simulink model "ModelAided_PAHRS"  (R2025b)
settings: Solver=ode4  StartTime=0.0  StopTime=300  RelTol=1e-3
values from neighbouring files (symbols this model uses):
  b_a = [0.090; -0.120; 0.075]    [Initilization.m]
  b_w = [-0.0009; 0.0010; -0.0015]    [Initilization.m]
  M_a = [50000, -15000, 10000;                   -7500, -60000, 12500;                  -12500,   5000, 20000] * 1E-6    [Initilization.m]
  M_w = [40000, -14000,  12500;                       0, -30000,  -7500;                       0,      0, -17500] * 1E-6    [Initilization.m]
libraries: slpidlib x16, simulink_extras x13, simulink x8, aerolibobsolete x4
(part 1 of 3)
settings Model: Creator=Arsinsoft  LastModifiedBy=Arsinsoft
settings OptimizationCC: ReuseModelBlockBuffer=off
settings RTWCC: GPUComputeCapability=3.5

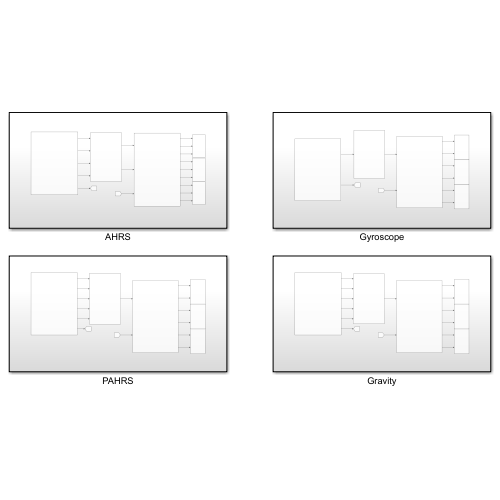
[thumbnail: Simulink's stored preview of the top-level diagram]
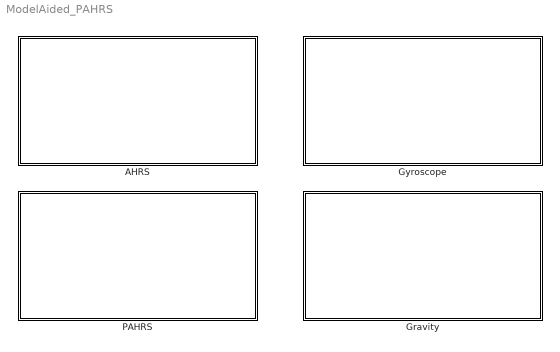
== system ModelAided_PAHRS ==
  AHRS : Subsystem
  Gravity : Subsystem
  Gyroscope : Subsystem
  PAHRS : Subsystem

== system ModelAided_PAHRS/AHRS ==
  AHRS (Euler - KF - Closed Loop) : Subsystem
  Dynamic Model : Subsystem
  Scope : Subsystem
  Scope1 : Scope  NumInputPorts=3
      settings: ActiveDisplayYMinimum=-4.56009  ActiveDisplayYMaximum=22.67075
  Scope2 : Scope  NumInputPorts=3
      settings: ActiveDisplayYMinimum=-2.66951  ActiveDisplayYMaximum=2.86704
  Scope3 : Scope  NumInputPorts=3
      settings: ActiveDisplayYMinimum=-8.24822  ActiveDisplayYMaximum=24.22827  DataLoggingVariableName=ScopeData2
  wires:
  Dynamic Model/4(psi_mes) -> AHRS (Euler - KF - Closed Loop)/4(psi_mes)
  Dynamic Model/3(a_B) -> AHRS (Euler - KF - Closed Loop)/3(a_B)
  Dynamic Model/2(f_B) -> AHRS (Euler - KF - Closed Loop)/2(f_B)
  Dynamic Model/1(omega_B) -> AHRS (Euler - KF - Closed Loop)/1(omega_B)
  AHRS (Euler - KF - Closed Loop)/1(xhat) -> Scope/1(xhat)
  AHRS (Euler - KF - Closed Loop)/2(y_mes) -> Scope/2(y_mes)
  Scope/1(phi_true) -> Scope1/1  "phi_true"
  Scope/2(phi_mes) -> Scope1/2  "phi_mes"
  Scope/3(phi_hat) -> Scope1/3  "phi_hat"
  Scope/5(theta_mes) -> Scope2/2  "theta_mes"
  Scope/4(theta_true) -> Scope2/1  "theta_true"
  Scope/6(theta_hat) -> Scope2/3  "theta_hat"
  Scope/7(psi_true) -> Scope3/1  "psi_true"
  Scope/8(psi_mes) -> Scope3/2  "psi_mes"
  Scope/9(psi_hat) -> Scope3/3  "psi_hat"
  Dynamic Model/5(A_true) -> [A_true]
  [A_true] -> Scope/3(A_true)

== system ModelAided_PAHRS/Gravity ==
  Dynamic Model : Subsystem
  PAHRS (Euler - KF - Closed Loop) : Subsystem
  Scope : Subsystem
  Scope1 : Scope  NumInputPorts=2
      settings: ActiveDisplayYMinimum=-22.604189397145177  ActiveDisplayYMaximum=33.93959392130872
  Scope2 : Scope  NumInputPorts=2
      settings: ActiveDisplayYMinimum=-1.1950277273773284  ActiveDisplayYMaximum=1.0982346892038803  DataLoggingVariableName=ScopeData4
  Scope3 : Scope  NumInputPorts=2
      settings: ActiveDisplayYMinimum=-16.246693349234917  ActiveDisplayYMaximum=108.31140694961906  DataLoggingVariableName=ScopeData3
  wires:
  Scope/6(psi_gravity) -> Scope3/2  "psi_gravity"
  PAHRS (Euler - KF - Closed Loop)/1(xhat) -> Scope/1(xhat)
  Scope/1(phi_true) -> Scope1/1  "phi_true"
  Scope/2(phi_gravity) -> Scope1/2  "phi_gravity"
  Scope/3(theta_true) -> Scope2/1  "theta_true"
  Scope/4(theta_gravity) -> Scope2/2  "theta_gravity"
  Scope/5(psi_true) -> Scope3/1  "psi_true"
  [A_true] -> Scope/2(A_true)
  Dynamic Model/6(A_true) -> [A_true]
  Dynamic Model/5(psi_mes2) -> PAHRS (Euler - KF - Closed Loop)/5(psi_mes2)
  Dynamic Model/4(psi_mes1) -> PAHRS (Euler - KF - Closed Loop)/4(psi_mes1)
  Dynamic Model/3(a_B) -> PAHRS (Euler - KF - Closed Loop)/3(a_B)
  Dynamic Model/1(omega_B) -> PAHRS (Euler - KF - Closed Loop)/1(omega_B)
  Dynamic Model/2(f_B) -> PAHRS (Euler - KF - Closed Loop)/2(f_B)

== system ModelAided_PAHRS/Gyroscope ==
  Dynamic Model : Subsystem
  Propagation : Subsystem
  Scope : Subsystem
  Scope1 : Scope  NumInputPorts=2
      settings: ActiveDisplayYMinimum=-37.126063824866776  ActiveDisplayYMaximum=33.465463609284008
  Scope2 : Scope  NumInputPorts=2
      settings: ActiveDisplayYMinimum=-7.2234114605205  ActiveDisplayYMaximum=39.031362224782178  DataLoggingVariableName=ScopeData4
  Scope3 : Scope  NumInputPorts=2
      settings: ActiveDisplayYMinimum=-34.052279453447049  ActiveDisplayYMaximum=109.90874054758552  DataLoggingVariableName=ScopeData3
  wires:
  [A_true] -> Scope/2(A_true)
  Scope/5(psi_true) -> Scope3/1  "psi_true"
  Scope/4(theta_gyro) -> Scope2/2  "theta_gyro"
  Scope/3(theta_true) -> Scope2/1  "theta_true"
  Scope/2(phi_gyro) -> Scope1/2  "phi_gyro"
  Scope/1(phi_true) -> Scope1/1  "phi_true"
  Propagation/1(x_gyro) -> Scope/1(x_gyro)
  Scope/6(psi_gyro) -> Scope3/2  "psi_gyro"
  Dynamic Model/1(omega_B) -> Propagation/1(omega_B)
  Dynamic Model/2(A_true) -> [A_true]

== system ModelAided_PAHRS/PAHRS ==
  Dynamic Model : Subsystem
  PAHRS (Euler - KF - Closed Loop) : Subsystem
  Scope : Subsystem
  Scope1 : Scope  NumInputPorts=2
      settings: ActiveDisplayYMinimum=-6.9171932251670389  ActiveDisplayYMaximum=31.887881688968882
  Scope2 : Scope  NumInputPorts=2
      settings: ActiveDisplayYMinimum=-1.1472184157024201  ActiveDisplayYMaximum=1.0928796557242522  DataLoggingVariableName=ScopeData4
  Scope3 : Scope  NumInputPorts=2
      settings: ActiveDisplayYMinimum=-16.332769192632206  ActiveDisplayYMaximum=108.42060570484539  DataLoggingVariableName=ScopeData3
  wires:
  [A_true] -> Scope/2(A_true)
  Scope/5(psi_true) -> Scope3/1  "psi_true"
  Scope/4(theta_hat) -> Scope2/2  "theta_hat"
  Scope/3(theta_true) -> Scope2/1  "theta_true"
  Scope/2(phi_hat) -> Scope1/2  "phi_hat"
  Scope/1(phi_true) -> Scope1/1  "phi_true"
  PAHRS (Euler - KF - Closed Loop)/1(xhat) -> Scope/1(xhat)
  Scope/6(psi_hat) -> Scope3/2  "psi_hat"
  Dynamic Model/6(A_true) -> [A_true]
  Dynamic Model/5(psi_mes2) -> PAHRS (Euler - KF - Closed Loop)/5(psi_mes2)
  Dynamic Model/4(psi_mes1) -> PAHRS (Euler - KF - Closed Loop)/4(psi_mes1)
  Dynamic Model/3(a_B) -> PAHRS (Euler - KF - Closed Loop)/3(a_B)
  Dynamic Model/2(f_B) -> PAHRS (Euler - KF - Closed Loop)/2(f_B)
  Dynamic Model/1(omega_B) -> PAHRS (Euler - KF - Closed Loop)/1(omega_B)

== system ModelAided_PAHRS/AHRS/AHRS (Euler - KF - Closed Loop) ==
  omega_B : Inport
  f_B : Inport  Port=2
  a_B : Inport  Port=3
  psi_mes : Inport  Port=4
  Clock : Clock
  Enable : MATLAB Function  TreatAsAtomicUnit=on
  KF : Subsystem  TreatAsAtomicUnit=on
  Measurement : Subsystem
  Propagation : Subsystem
  Sum : Sum  Inputs=++|
  xhat : Outport
  y_mes : Outport  Port=2
  wires:
  Propagation/1(x_prop) -> KF/2(x_prop), Sum/1  "x_prop"
  Measurement/1(y_mes) -> y_mes/1, KF/3(y_mes)  "y_mes"
  KF/1(deltaxhat) -> Sum/2
  Enable/1(enable) -> KF/Enable
  Sum/1 -> Propagation/2(xhat), xhat/1
  Clock/1 -> Enable/1(t)
  omega_B/1 -> KF/1(omega_B), Propagation/1(omega_B)
  f_B/1 -> Measurement/2(f_B)
  a_B/1 -> Measurement/1(a_B)
  psi_mes/1 -> Measurement/3(psi_mes)

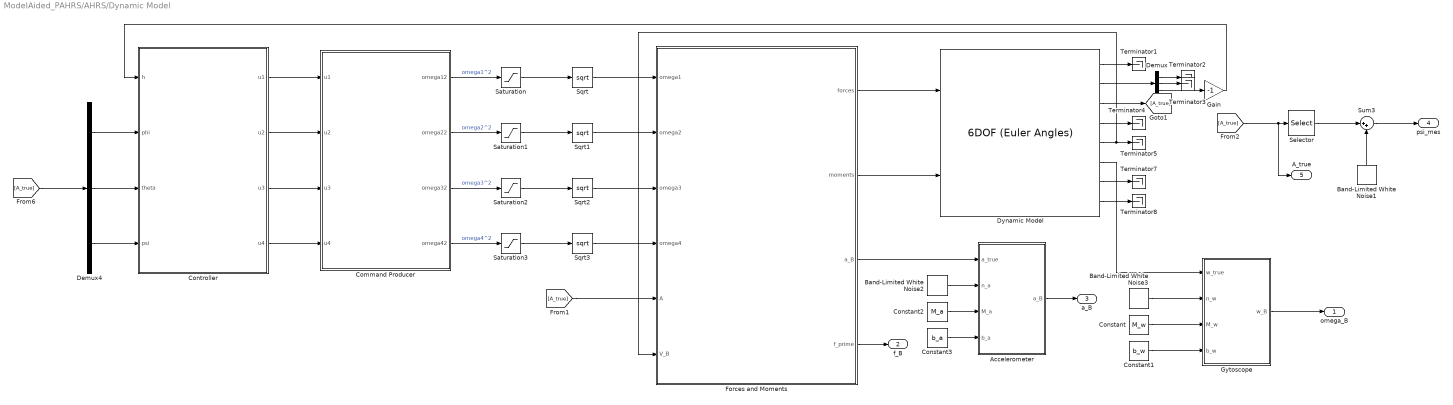
== system ModelAided_PAHRS/AHRS/Dynamic Model ==
  Accelerometer : MATLAB Function  TreatAsAtomicUnit=on
  Band-Limited White Noise1 : simulink/Sources/Band-Limited White Noise  Cov=1e-5  Ts=0.01  seed=[23341]
  Band-Limited White Noise2 : simulink/Sources/Band-Limited White Noise  Cov=1e-4  Ts=0.01  seed=[23341]
  Band-Limited White Noise3 : simulink/Sources/Band-Limited White Noise  Cov=1e-4  Ts=0.01  seed=[23341]
  Command Producer : MATLAB Function  TreatAsAtomicUnit=on
  Constant : Constant  Value=M_w
  Constant1 : Constant  Value=b_w
  Constant2 : Constant  Value=M_a
  Constant3 : Constant  Value=b_a
  Controller : Subsystem
  Demux : Demux  Outputs=3
  Demux4 : Demux  Outputs=3
  Dynamic Model : aerolibobsolete/6DOF (Euler Angles)  units=Metric (MKS)  mtype=Fixed  rep=Euler Angles  xme_0=[0 0 0]  Vm_0=[0 0 0]  eul_0=[0 0 0]  pm_0=[0 0 0]  mass_0=0.296  mass_e=0.5  mass_f=2.0  inertia=[0.0049, 0, 0; 0, 0.0049, 0; 0, 0, 0.0088]  inertia_e=eye(3)  inertia_f=2*eye(3)  k_quat=1.0  vre_flag=on  abi_flag=off  aMode=0  xme_statename=''  Vm_statename=''  eul_statename=''  quat_statename=''  pm_statename=''  mass_statename=''
  Forces and Moments : MATLAB Function  TreatAsAtomicUnit=on
  Gain : Gain  Gain=-1
  Gytoscope : MATLAB Function  TreatAsAtomicUnit=on
  Saturation{,1..3} (4 alike) : Saturate  UpperLimit=7e6  LowerLimit=138e3
  Selector : Selector  InputPortWidth=3  IndexOptions=Index vector (dialog)  Indices=[3]  OutputSizes=1
  Sqrt{,1..3} (4 alike) : Sqrt
  Sum3 : Sum  Inputs=|++
  Terminator{1..5,7..8} (7 alike) : Terminator
  omega_B : Outport
  f_B : Outport  Port=2
  a_B : Outport  Port=3
  psi_mes : Outport  Port=4
  A_true : Outport  Port=5
  wires:
  Forces and Moments/2(moments) -> Dynamic Model/2
  Forces and Moments/1(forces) -> Dynamic Model/1
  Sum3/1 -> psi_mes/1
  Dynamic Model/1 -> Terminator1/1
  Dynamic Model/3 -> [A_true]
  Dynamic Model/4 -> Terminator4/1
  Dynamic Model/7 -> Terminator7/1
  Dynamic Model/8 -> Terminator8/1
  Dynamic Model/5 -> Terminator5/1, Forces and Moments/6(V_B)
  Band-Limited White Noise1/1 -> Sum3/2
  Selector/1 -> Sum3/1
  [A_true] -> Forces and Moments/5(A)
  [A_true] -> A_true/1, Selector/1
  Dynamic Model/6 -> Gytoscope/1(w_true)
  [A_true] -> Demux4/1
  Demux4/3 -> Controller/4(psi)
  Demux4/2 -> Controller/3(theta)
  Demux4/1 -> Controller/2(phi)
  Command Producer/2(omega22) -> Saturation1/1  "omega2^2"
  Controller/1(u1) -> Command Producer/1(u1)
  Controller/3(u3) -> Command Producer/3(u3)
  Command Producer/4(omega42) -> Saturation3/1  "omega4^2"
  Saturation/1 -> Sqrt/1
  Controller/4(u4) -> Command Producer/4(u4)
  Saturation3/1 -> Sqrt3/1
  Command Producer/1(omega12) -> Saturation/1  "omega1^2"
  Command Producer/3(omega32) -> Saturation2/1  "omega3^2"
  Saturation2/1 -> Sqrt2/1
  Controller/2(u2) -> Command Producer/2(u2)
  Saturation1/1 -> Sqrt1/1
  Sqrt/1 -> Forces and Moments/1(omega1)
  Sqrt1/1 -> Forces and Moments/2(omega2)
  Sqrt2/1 -> Forces and Moments/3(omega3)
  Sqrt3/1 -> Forces and Moments/4(omega4)
  Dynamic Model/2 -> Demux/1
  Demux/1 -> Terminator2/1
  Demux/2 -> Terminator3/1
  Demux/3 -> Gain/1
  Gain/1 -> Controller/1(h)
  Forces and Moments/4(f_prime) -> f_B/1
  Accelerometer/1(a_B) -> a_B/1
  Forces and Moments/3(a_B) -> Accelerometer/1(a_true)
  Band-Limited White Noise2/1 -> Accelerometer/2(n_a)
  Band-Limited White Noise3/1 -> Gytoscope/2(n_w)
  Gytoscope/1(w_B) -> omega_B/1
  Constant/1 -> Gytoscope/3(M_w)
  Constant1/1 -> Gytoscope/4(b_w)
  Constant3/1 -> Accelerometer/4(b_a)
  Constant2/1 -> Accelerometer/3(M_a)

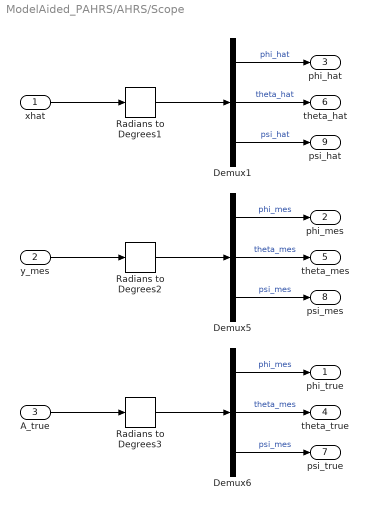
== system ModelAided_PAHRS/AHRS/Scope ==
  xhat : Inport
  y_mes : Inport  Port=2
  A_true : Inport  Port=3
  Demux1 : Demux  Outputs=3
  Demux5 : Demux  Outputs=3
  Demux6 : Demux  Outputs=3
  Radians to Degrees1 : simulink_extras/Transformations/Radians to Degrees
  Radians to Degrees2 : simulink_extras/Transformations/Radians to Degrees
  Radians to Degrees3 : simulink_extras/Transformations/Radians to Degrees
  phi_true : Outport
  phi_mes : Outport  Port=2
  phi_hat : Outport  Port=3
  theta_true : Outport  Port=4
  theta_mes : Outport  Port=5
  theta_hat : Outport  Port=6
  psi_true : Outport  Port=7
  psi_mes : Outport  Port=8
  psi_hat : Outport  Port=9
  wires:
  Demux1/2 -> theta_hat/1  "theta_hat"
  Demux1/3 -> psi_hat/1  "psi_hat"
  Demux1/1 -> phi_hat/1  "phi_hat"
  xhat/1 -> Radians to Degrees1/1
  Radians to Degrees1/1 -> Demux1/1
  Radians to Degrees2/1 -> Demux5/1
  Demux5/1 -> phi_mes/1  "phi_mes"
  Demux5/3 -> psi_mes/1  "psi_mes"
  Demux5/2 -> theta_mes/1  "theta_mes"
  y_mes/1 -> Radians to Degrees2/1
  Demux6/2 -> theta_true/1  "theta_mes"
  Demux6/3 -> psi_true/1  "psi_mes"
  Demux6/1 -> phi_true/1  "phi_mes"
  Radians to Degrees3/1 -> Demux6/1
  A_true/1 -> Radians to Degrees3/1

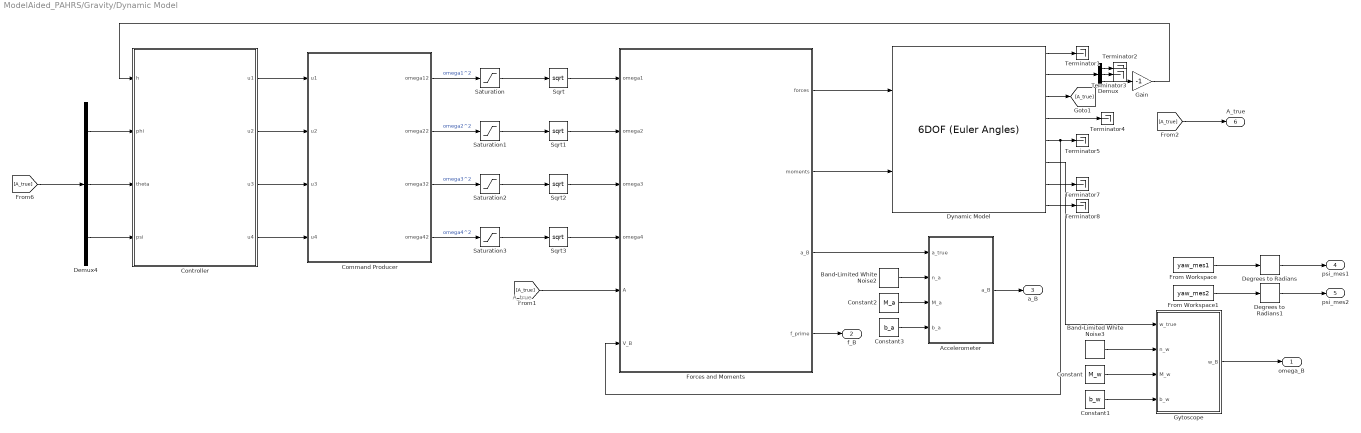
== system ModelAided_PAHRS/Gravity/Dynamic Model ==
  note: A_true
  Accelerometer : MATLAB Function  TreatAsAtomicUnit=on
  Band-Limited White Noise2 : simulink/Sources/Band-Limited White Noise  Cov=1e-4  Ts=0.01  seed=[23341]
  Band-Limited White Noise3 : simulink/Sources/Band-Limited White Noise  Cov=1e-4  Ts=0.01  seed=[23341]
  Command Producer : MATLAB Function  TreatAsAtomicUnit=on
  Constant : Constant  Value=M_w
  Constant1 : Constant  Value=b_w
  Constant2 : Constant  Value=M_a
  Constant3 : Constant  Value=b_a
  Controller : Subsystem
  Degrees to Radians : simulink_extras/Transformations/Degrees to Radians
  Degrees to Radians1 : simulink_extras/Transformations/Degrees to Radians
  Demux : Demux  Outputs=3
  Demux4 : Demux  Outputs=3
  Dynamic Model : aerolibobsolete/6DOF (Euler Angles)  units=Metric (MKS)  mtype=Fixed  rep=Euler Angles  xme_0=[0 0 -10]  Vm_0=[0 0 0]  eul_0=[0 0 0]  pm_0=[0 0 0]  mass_0=0.296  mass_e=0.5  mass_f=2.0  inertia=[0.0049, 0, 0; 0, 0.0049, 0; 0, 0, 0.0088]  inertia_e=eye(3)  inertia_f=2*eye(3)  k_quat=1.0  vre_flag=on  abi_flag=off  aMode=0  xme_statename=''  Vm_statename=''  eul_statename=''  quat_statename=''  pm_statename=''  mass_statename=''
  Forces and Moments : MATLAB Function  TreatAsAtomicUnit=on
  From Workspace : FromWorkspace  VariableName=yaw_mes1  OutDataTypeStr=double  SampleTime=-1  Interpolate=off  OutputAfterFinalValue=Holding final value
  From Workspace1 : FromWorkspace  VariableName=yaw_mes2  OutDataTypeStr=double  SampleTime=-1  Interpolate=off  OutputAfterFinalValue=Holding final value
  Gain : Gain  Gain=-1
  Gytoscope : MATLAB Function  TreatAsAtomicUnit=on
  Saturation{,1..3} (4 alike) : Saturate  UpperLimit=7e6  LowerLimit=138e3
  Sqrt{,1..3} (4 alike) : Sqrt
  Terminator{1..5,7..8} (7 alike) : Terminator
  omega_B : Outport
  f_B : Outport  Port=2
  a_B : Outport  Port=3
  psi_mes1 : Outport  Port=4
  psi_mes2 : Outport  Port=5
  A_true : Outport  Port=6
  wires:
  Gain/1 -> Controller/1(h)
  [A_true] -> Demux4/1
  Demux4/3 -> Controller/4(psi)
  Demux4/1 -> Controller/2(phi)
  Demux4/2 -> Controller/3(theta)
  Demux/3 -> Gain/1
  Demux/2 -> Terminator3/1
  Demux/1 -> Terminator2/1
  Sqrt3/1 -> Forces and Moments/4(omega4)
  Saturation2/1 -> Sqrt2/1
  Controller/1(u1) -> Command Producer/1(u1)
  Controller/3(u3) -> Command Producer/3(u3)
  Command Producer/4(omega42) -> Saturation3/1  "omega4^2"
  Command Producer/2(omega22) -> Saturation1/1  "omega2^2"
  Saturation/1 -> Sqrt/1
  Controller/2(u2) -> Command Producer/2(u2)
  Command Producer/3(omega32) -> Saturation2/1  "omega3^2"
  Command Producer/1(omega12) -> Saturation/1  "omega1^2"
  Controller/4(u4) -> Command Producer/4(u4)
  Saturation3/1 -> Sqrt3/1
  Saturation1/1 -> Sqrt1/1
  Forces and Moments/2(moments) -> Dynamic Model/2
  Forces and Moments/1(forces) -> Dynamic Model/1
  Dynamic Model/1 -> Terminator1/1
  Dynamic Model/2 -> Demux/1
  Dynamic Model/3 -> [A_true]
  Dynamic Model/4 -> Terminator4/1
  Dynamic Model/7 -> Terminator7/1
  Dynamic Model/8 -> Terminator8/1
  Dynamic Model/5 -> Terminator5/1, Forces and Moments/6(V_B)
  [A_true] -> Forces and Moments/5(A)
  [A_true] -> A_true/1
  Sqrt2/1 -> Forces and Moments/3(omega3)
  Sqrt1/1 -> Forces and Moments/2(omega2)
  Sqrt/1 -> Forces and Moments/1(omega1)
  Forces and Moments/4(f_prime) -> f_B/1
  Degrees to Radians1/1 -> psi_mes2/1
  From Workspace/1 -> Degrees to Radians/1
  From Workspace1/1 -> Degrees to Radians1/1
  Degrees to Radians/1 -> psi_mes1/1
  Gytoscope/1(w_B) -> omega_B/1
  Constant3/1 -> Accelerometer/4(b_a)
  Constant2/1 -> Accelerometer/3(M_a)
  Band-Limited White Noise2/1 -> Accelerometer/2(n_a)
  Forces and Moments/3(a_B) -> Accelerometer/1(a_true)
  Accelerometer/1(a_B) -> a_B/1
  Constant1/1 -> Gytoscope/4(b_w)
  Constant/1 -> Gytoscope/3(M_w)
  Band-Limited White Noise3/1 -> Gytoscope/2(n_w)
  Dynamic Model/6 -> Gytoscope/1(w_true)

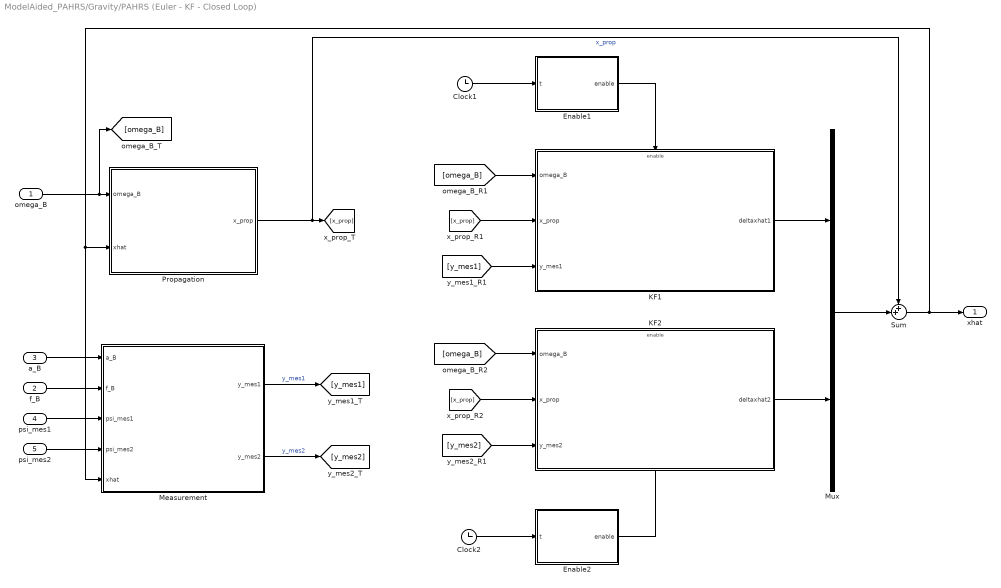
== system ModelAided_PAHRS/Gravity/PAHRS (Euler - KF - Closed Loop) ==
  omega_B : Inport
  f_B : Inport  Port=2
  a_B : Inport  Port=3
  psi_mes1 : Inport  Port=4
  psi_mes2 : Inport  Port=5
  Clock1 : Clock
  Clock2 : Clock
  Enable1 : MATLAB Function  TreatAsAtomicUnit=on
  Enable2 : MATLAB Function  TreatAsAtomicUnit=on
  KF1 : Subsystem  TreatAsAtomicUnit=on
  KF2 : Subsystem  TreatAsAtomicUnit=on
  Measurement : Subsystem
  Mux : Mux  Inputs=2
  Propagation : Subsystem
  Sum : Sum  Inputs=++|
  xhat : Outport
  wires:
  KF2/1(deltaxhat2) -> Mux/2
  Mux/1 -> Sum/2
  KF1/1(deltaxhat1) -> Mux/1
  Enable1/1(enable) -> KF1/Enable
  Enable2/1(enable) -> KF2/Enable
  Clock2/1 -> Enable2/1(t)
  [y_mes2] -> KF2/3(y_mes2)
  [y_mes1] -> KF1/3(y_mes1)
  [omega_B] -> KF2/1(omega_B)
  [omega_B] -> KF1/1(omega_B)
  [x_prop] -> KF2/2(x_prop)
  [x_prop] -> KF1/2(x_prop)
  Propagation/1(x_prop) -> [x_prop], Sum/1  "x_prop"
  Clock1/1 -> Enable1/1(t)
  omega_B/1 -> Propagation/1(omega_B), [omega_B]
  Sum/1 -> xhat/1, Propagation/2(xhat), Measurement/5(xhat)
  psi_mes2/1 -> Measurement/4(psi_mes2)
  Measurement/1(y_mes1) -> [y_mes1]  "y_mes1"
  f_B/1 -> Measurement/2(f_B)
  Measurement/2(y_mes2) -> [y_mes2]  "y_mes2"
  psi_mes1/1 -> Measurement/3(psi_mes1)
  a_B/1 -> Measurement/1(a_B)

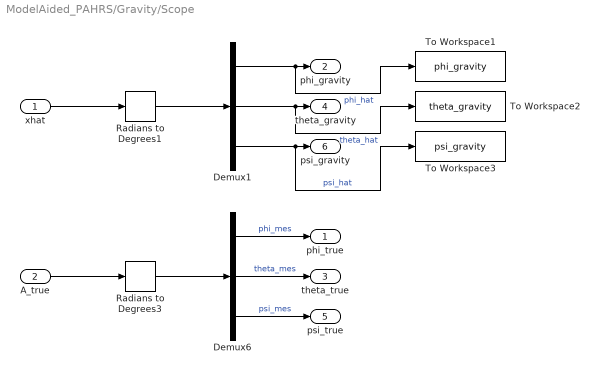
== system ModelAided_PAHRS/Gravity/Scope ==
  xhat : Inport
  A_true : Inport  Port=2
  Demux1 : Demux  Outputs=3
  Demux6 : Demux  Outputs=3
  Radians to Degrees1 : simulink_extras/Transformations/Radians to Degrees
  Radians to Degrees3 : simulink_extras/Transformations/Radians to Degrees
  To Workspace1 : ToWorkspace  VariableName=phi_gravity  SampleTime=-1
      settings: Save2DSignal=2-D array (concatenate along first dimension)
  To Workspace2 : ToWorkspace  VariableName=theta_gravity  SampleTime=-1
      settings: Save2DSignal=2-D array (concatenate along first dimension)
  To Workspace3 : ToWorkspace  VariableName=psi_gravity  SampleTime=-1
      settings: Save2DSignal=2-D array (concatenate along first dimension)
  phi_true : Outport
  phi_gravity : Outport  Port=2
  theta_true : Outport  Port=3
  theta_gravity : Outport  Port=4
  psi_true : Outport  Port=5
  psi_gravity : Outport  Port=6
  wires:
  Demux1/2 -> theta_gravity/1, To Workspace2/1  "theta_hat"
  Demux1/3 -> psi_gravity/1, To Workspace3/1  "psi_hat"
  Demux1/1 -> phi_gravity/1, To Workspace1/1  "phi_hat"
  xhat/1 -> Radians to Degrees1/1
  Radians to Degrees1/1 -> Demux1/1
  Demux6/2 -> theta_true/1  "theta_mes"
  Demux6/3 -> psi_true/1  "psi_mes"
  Demux6/1 -> phi_true/1  "phi_mes"
  Radians to Degrees3/1 -> Demux6/1
  A_true/1 -> Radians to Degrees3/1

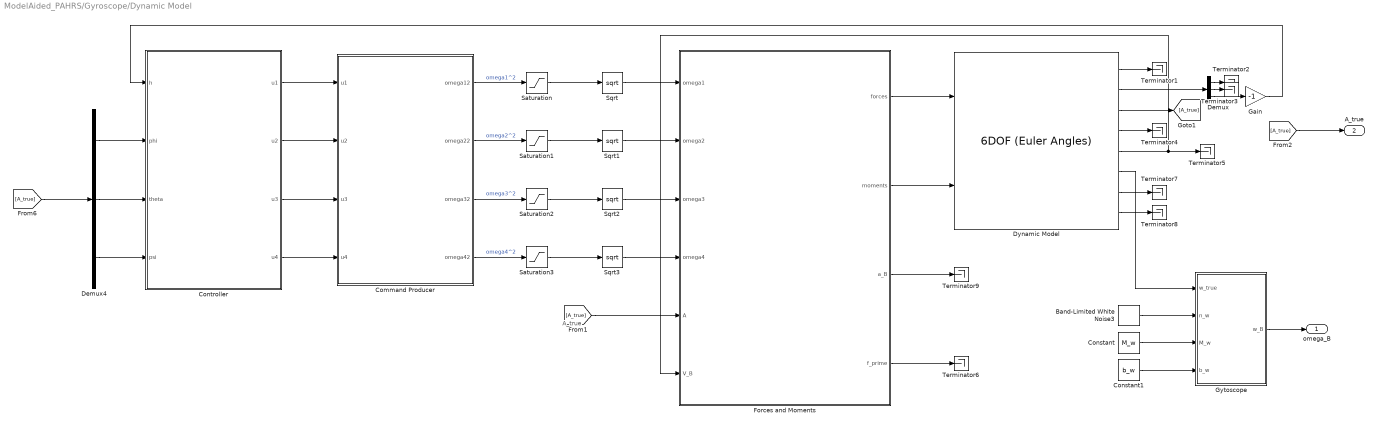
== system ModelAided_PAHRS/Gyroscope/Dynamic Model ==
  note: A_true
  Band-Limited White Noise3 : simulink/Sources/Band-Limited White Noise  Cov=1e-4  Ts=0.01  seed=[23341]
  Command Producer : MATLAB Function  TreatAsAtomicUnit=on
  Constant : Constant  Value=M_w
  Constant1 : Constant  Value=b_w
  Controller : Subsystem
  Demux : Demux  Outputs=3
  Demux4 : Demux  Outputs=3
  Dynamic Model : aerolibobsolete/6DOF (Euler Angles)  units=Metric (MKS)  mtype=Fixed  rep=Euler Angles  xme_0=[0 0 -10]  Vm_0=[0 0 0]  eul_0=[0 0 0]  pm_0=[0 0 0]  mass_0=0.296  mass_e=0.5  mass_f=2.0  inertia=[0.0049, 0, 0; 0, 0.0049, 0; 0, 0, 0.0088]  inertia_e=eye(3)  inertia_f=2*eye(3)  k_quat=1.0  vre_flag=on  abi_flag=off  aMode=0  xme_statename=''  Vm_statename=''  eul_statename=''  quat_statename=''  pm_statename=''  mass_statename=''
  Forces and Moments : MATLAB Function  TreatAsAtomicUnit=on
  Gain : Gain  Gain=-1
  Gytoscope : MATLAB Function  TreatAsAtomicUnit=on
  Saturation{,1..3} (4 alike) : Saturate  UpperLimit=7e6  LowerLimit=138e3
  Sqrt{,1..3} (4 alike) : Sqrt
  Terminator{1..9} (9 alike) : Terminator
  omega_B : Outport
  A_true : Outport  Port=2
  wires:
  Sqrt/1 -> Forces and Moments/1(omega1)
  Sqrt1/1 -> Forces and Moments/2(omega2)
  Sqrt2/1 -> Forces and Moments/3(omega3)
  [A_true] -> A_true/1
  [A_true] -> Forces and Moments/5(A)
  Dynamic Model/5 -> Terminator5/1, Forces and Moments/6(V_B)
  Dynamic Model/8 -> Terminator8/1
  Dynamic Model/7 -> Terminator7/1
  Dynamic Model/4 -> Terminator4/1
  Dynamic Model/3 -> [A_true]
  Dynamic Model/2 -> Demux/1
  Dynamic Model/1 -> Terminator1/1
  Forces and Moments/1(forces) -> Dynamic Model/1
  Forces and Moments/2(moments) -> Dynamic Model/2
  Saturation1/1 -> Sqrt1/1
  Saturation3/1 -> Sqrt3/1
  Controller/4(u4) -> Command Producer/4(u4)
  Command Producer/1(omega12) -> Saturation/1  "omega1^2"
  Command Producer/3(omega32) -> Saturation2/1  "omega3^2"
  Controller/2(u2) -> Command Producer/2(u2)
  Saturation/1 -> Sqrt/1
  Command Producer/2(omega22) -> Saturation1/1  "omega2^2"
  Command Producer/4(omega42) -> Saturation3/1  "omega4^2"
  Controller/3(u3) -> Command Producer/3(u3)
  Controller/1(u1) -> Command Producer/1(u1)
  Saturation2/1 -> Sqrt2/1
  Sqrt3/1 -> Forces and Moments/4(omega4)
  Demux/1 -> Terminator2/1
  Demux/2 -> Terminator3/1
  Demux/3 -> Gain/1
  Demux4/2 -> Controller/3(theta)
  Demux4/1 -> Controller/2(phi)
  Demux4/3 -> Controller/4(psi)
  [A_true] -> Demux4/1
  Gain/1 -> Controller/1(h)
  Forces and Moments/3(a_B) -> Terminator9/1
  Forces and Moments/4(f_prime) -> Terminator6/1
  Constant1/1 -> Gytoscope/4(b_w)
  Constant/1 -> Gytoscope/3(M_w)
  Band-Limited White Noise3/1 -> Gytoscope/2(n_w)
  Dynamic Model/6 -> Gytoscope/1(w_true)
  Gytoscope/1(w_B) -> omega_B/1

== system ModelAided_PAHRS/Gyroscope/Propagation ==
  omega_B : Inport
  Propagation1 : MATLAB Function  TreatAsAtomicUnit=on
  Unit Delay : UnitDelay  InitialCondition=[0;0;0]  SampleTime=-1  HasFrameUpgradeWarning=on
  x_gyro : Outport
  wires:
  Propagation1/1(A_prop) -> Unit Delay/1, x_gyro/1
  omega_B/1 -> Propagation1/1(omega_B)
  Unit Delay/1 -> Propagation1/2(A_prev)

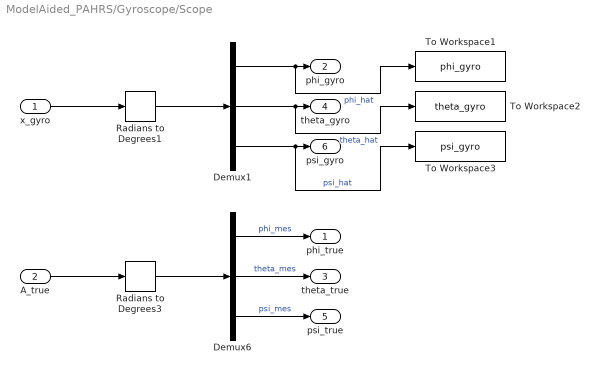
== system ModelAided_PAHRS/Gyroscope/Scope ==
  x_gyro : Inport
  A_true : Inport  Port=2
  Demux1 : Demux  Outputs=3
  Demux6 : Demux  Outputs=3
  Radians to Degrees1 : simulink_extras/Transformations/Radians to Degrees
  Radians to Degrees3 : simulink_extras/Transformations/Radians to Degrees
  To Workspace1 : ToWorkspace  VariableName=phi_gyro  SampleTime=-1
      settings: Save2DSignal=2-D array (concatenate along first dimension)
  To Workspace2 : ToWorkspace  VariableName=theta_gyro  SampleTime=-1
      settings: Save2DSignal=2-D array (concatenate along first dimension)
  To Workspace3 : ToWorkspace  VariableName=psi_gyro  SampleTime=-1
      settings: Save2DSignal=2-D array (concatenate along first dimension)
  phi_true : Outport
  phi_gyro : Outport  Port=2
  theta_true : Outport  Port=3
  theta_gyro : Outport  Port=4
  psi_true : Outport  Port=5
  psi_gyro : Outport  Port=6
  wires:
  A_true/1 -> Radians to Degrees3/1
  Radians to Degrees3/1 -> Demux6/1
  Demux6/1 -> phi_true/1  "phi_mes"
  Demux6/3 -> psi_true/1  "psi_mes"
  Demux6/2 -> theta_true/1  "theta_mes"
  Radians to Degrees1/1 -> Demux1/1
  x_gyro/1 -> Radians to Degrees1/1
  Demux1/1 -> To Workspace1/1, phi_gyro/1  "phi_hat"
  Demux1/3 -> To Workspace3/1, psi_gyro/1  "psi_hat"
  Demux1/2 -> To Workspace2/1, theta_gyro/1  "theta_hat"

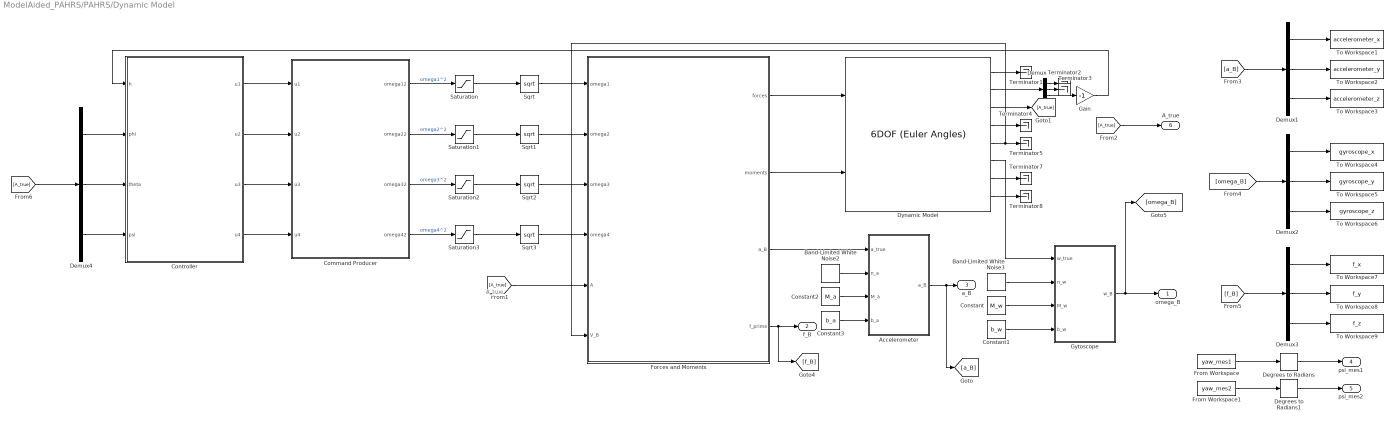
== system ModelAided_PAHRS/PAHRS/Dynamic Model ==
  note: A_true
  Accelerometer : MATLAB Function  TreatAsAtomicUnit=on
  Band-Limited White Noise2 : simulink/Sources/Band-Limited White Noise  Cov=1e-4  Ts=0.01  seed=[23341]
  Band-Limited White Noise3 : simulink/Sources/Band-Limited White Noise  Cov=1e-4  Ts=0.01  seed=[23341]
  Command Producer : MATLAB Function  TreatAsAtomicUnit=on
  Constant : Constant  Value=M_w
  Constant1 : Constant  Value=b_w
  Constant2 : Constant  Value=M_a
  Constant3 : Constant  Value=b_a
  Controller : Subsystem
  Degrees to Radians : simulink_extras/Transformations/Degrees to Radians
  Degrees to Radians1 : simulink_extras/Transformations/Degrees to Radians
  Demux{,1..4} (5 alike) : Demux  Outputs=3
  Dynamic Model : aerolibobsolete/6DOF (Euler Angles)  units=Metric (MKS)  mtype=Fixed  rep=Euler Angles  xme_0=[0 0 -10]  Vm_0=[0 0 0]  eul_0=[0 0 0]  pm_0=[0 0 0]  mass_0=0.296  mass_e=0.5  mass_f=2.0  inertia=[0.0049, 0, 0; 0, 0.0049, 0; 0, 0, 0.0088]  inertia_e=eye(3)  inertia_f=2*eye(3)  k_quat=1.0  vre_flag=on  abi_flag=off  aMode=0  xme_statename=''  Vm_statename=''  eul_statename=''  quat_statename=''  pm_statename=''  mass_statename=''
  Forces and Moments : MATLAB Function  TreatAsAtomicUnit=on
  From Workspace : FromWorkspace  VariableName=yaw_mes1  OutDataTypeStr=double  SampleTime=-1  Interpolate=off  OutputAfterFinalValue=Holding final value
  From Workspace1 : FromWorkspace  VariableName=yaw_mes2  OutDataTypeStr=double  SampleTime=-1  Interpolate=off  OutputAfterFinalValue=Holding final value
  Gain : Gain  Gain=-1
  Gytoscope : MATLAB Function  TreatAsAtomicUnit=on
  Saturation{,1..3} (4 alike) : Saturate  UpperLimit=7e6  LowerLimit=138e3
  Sqrt{,1..3} (4 alike) : Sqrt
  Terminator{1..5,7..8} (7 alike) : Terminator
  To Workspace1 : ToWorkspace  VariableName=accelerometer_x  SampleTime=-1
      settings: Save2DSignal=2-D array (concatenate along first dimension)
  To Workspace2 : ToWorkspace  VariableName=accelerometer_y  SampleTime=-1
      settings: Save2DSignal=2-D array (concatenate along first dimension)
  To Workspace3 : ToWorkspace  VariableName=accelerometer_z  SampleTime=-1
      settings: Save2DSignal=2-D array (concatenate along first dimension)
  To Workspace4 : ToWorkspace  VariableName=gyroscope_x  SampleTime=-1
      settings: Save2DSignal=2-D array (concatenate along first dimension)
  To Workspace5 : ToWorkspace  VariableName=gyroscope_y  SampleTime=-1
      settings: Save2DSignal=2-D array (concatenate along first dimension)
  To Workspace6 : ToWorkspace  VariableName=gyroscope_z  SampleTime=-1
      settings: Save2DSignal=2-D array (concatenate along first dimension)
  To Workspace7 : ToWorkspace  VariableName=f_x  SampleTime=-1
      settings: Save2DSignal=2-D array (concatenate along first dimension)
  To Workspace8 : ToWorkspace  VariableName=f_y  SampleTime=-1
      settings: Save2DSignal=2-D array (concatenate along first dimension)
  To Workspace9 : ToWorkspace  VariableName=f_z  SampleTime=-1
      settings: Save2DSignal=2-D array (concatenate along first dimension)
  omega_B : Outport
  f_B : Outport  Port=2
  a_B : Outport  Port=3
  psi_mes1 : Outport  Port=4
  psi_mes2 : Outport  Port=5
  A_true : Outport  Port=6
  wires:
  Sqrt/1 -> Forces and Moments/1(omega1)
  Sqrt1/1 -> Forces and Moments/2(omega2)
  Sqrt2/1 -> Forces and Moments/3(omega3)
  [A_true] -> A_true/1
  [A_true] -> Forces and Moments/5(A)
  Dynamic Model/5 -> Forces and Moments/6(V_B), Terminator5/1
  Dynamic Model/8 -> Terminator8/1
  Dynamic Model/7 -> Terminator7/1
  Dynamic Model/4 -> Terminator4/1
  Dynamic Model/3 -> [A_true]
  Dynamic Model/2 -> Demux/1
  Dynamic Model/1 -> Terminator1/1
  Forces and Moments/1(forces) -> Dynamic Model/1
  Forces and Moments/2(moments) -> Dynamic Model/2
  From Workspace/1 -> Degrees to Radians/1
  Degrees to Radians/1 -> psi_mes1/1
  [a_B] -> Demux1/1
  Demux1/1 -> To Workspace1/1
  Demux1/2 -> To Workspace2/1
  Demux1/3 -> To Workspace3/1
  Demux2/3 -> To Workspace6/1
  Demux2/2 -> To Workspace5/1
  Demux2/1 -> To Workspace4/1
  [omega_B] -> Demux2/1
  [f_B] -> Demux3/1
  Demux3/1 -> To Workspace7/1
  Demux3/2 -> To Workspace8/1
  Demux3/3 -> To Workspace9/1
  Saturation1/1 -> Sqrt1/1
  Saturation3/1 -> Sqrt3/1
  Controller/4(u4) -> Command Producer/4(u4)
  Command Producer/1(omega12) -> Saturation/1  "omega1^2"
  Command Producer/3(omega32) -> Saturation2/1  "omega3^2"
  Controller/2(u2) -> Command Producer/2(u2)
  Saturation/1 -> Sqrt/1
  Command Producer/2(omega22) -> Saturation1/1  "omega2^2"
  Command Producer/4(omega42) -> Saturation3/1  "omega4^2"
  Controller/3(u3) -> Command Producer/3(u3)
  Controller/1(u1) -> Command Producer/1(u1)
  Saturation2/1 -> Sqrt2/1
  Sqrt3/1 -> Forces and Moments/4(omega4)
  Demux/1 -> Terminator2/1
  Demux/2 -> Terminator3/1
  Demux/3 -> Gain/1
  Demux4/2 -> Controller/3(theta)
  Demux4/1 -> Controller/2(phi)
  Demux4/3 -> Controller/4(psi)
  [A_true] -> Demux4/1
  Gain/1 -> Controller/1(h)
  Forces and Moments/4(f_prime) -> f_B/1, [f_B]
  Degrees to Radians1/1 -> psi_mes2/1
  From Workspace1/1 -> Degrees to Radians1/1
  Accelerometer/1(a_B) -> [a_B], a_B/1
  Constant3/1 -> Accelerometer/4(b_a)
  Constant2/1 -> Accelerometer/3(M_a)
  Band-Limited White Noise2/1 -> Accelerometer/2(n_a)
  Forces and Moments/3(a_B) -> Accelerometer/1(a_true)
  Constant1/1 -> Gytoscope/4(b_w)
  Constant/1 -> Gytoscope/3(M_w)
  Band-Limited White Noise3/1 -> Gytoscope/2(n_w)
  Dynamic Model/6 -> Gytoscope/1(w_true)
  Gytoscope/1(w_B) -> omega_B/1, [omega_B]

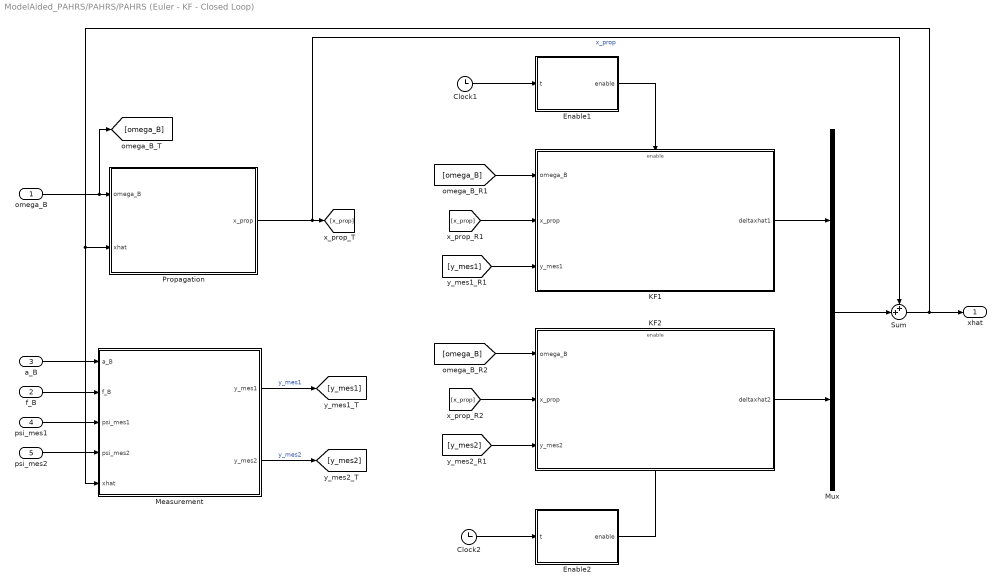
== system ModelAided_PAHRS/PAHRS/PAHRS (Euler - KF - Closed Loop) ==
  omega_B : Inport
  f_B : Inport  Port=2
  a_B : Inport  Port=3
  psi_mes1 : Inport  Port=4
  psi_mes2 : Inport  Port=5
  Clock1 : Clock
  Clock2 : Clock
  Enable1 : MATLAB Function  TreatAsAtomicUnit=on
  Enable2 : MATLAB Function  TreatAsAtomicUnit=on
  KF1 : Subsystem  TreatAsAtomicUnit=on
  KF2 : Subsystem  TreatAsAtomicUnit=on
  Measurement : Subsystem
  Mux : Mux  Inputs=2
  Propagation : Subsystem
  Sum : Sum  Inputs=++|
  xhat : Outport
  wires:
  psi_mes1/1 -> Measurement/3(psi_mes1)
  a_B/1 -> Measurement/1(a_B)
  f_B/1 -> Measurement/2(f_B)
  omega_B/1 -> [omega_B], Propagation/1(omega_B)
  Clock1/1 -> Enable1/1(t)
  Sum/1 -> Measurement/5(xhat), Propagation/2(xhat), xhat/1
  Propagation/1(x_prop) -> Sum/1, [x_prop]  "x_prop"
  Measurement/1(y_mes1) -> [y_mes1]  "y_mes1"
  Measurement/2(y_mes2) -> [y_mes2]  "y_mes2"
  [x_prop] -> KF1/2(x_prop)
  [x_prop] -> KF2/2(x_prop)
  [omega_B] -> KF1/1(omega_B)
  [omega_B] -> KF2/1(omega_B)
  [y_mes1] -> KF1/3(y_mes1)
  [y_mes2] -> KF2/3(y_mes2)
  Clock2/1 -> Enable2/1(t)
  Enable2/1(enable) -> KF2/Enable
  Enable1/1(enable) -> KF1/Enable
  KF1/1(deltaxhat1) -> Mux/1
  Mux/1 -> Sum/2
  KF2/1(deltaxhat2) -> Mux/2
  psi_mes2/1 -> Measurement/4(psi_mes2)

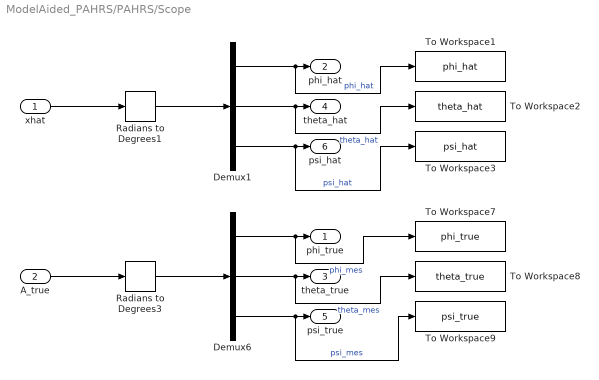
== system ModelAided_PAHRS/PAHRS/Scope ==
  xhat : Inport
  A_true : Inport  Port=2
  Demux1 : Demux  Outputs=3
  Demux6 : Demux  Outputs=3
  Radians to Degrees1 : simulink_extras/Transformations/Radians to Degrees
  Radians to Degrees3 : simulink_extras/Transformations/Radians to Degrees
  To Workspace1 : ToWorkspace  VariableName=phi_hat  SampleTime=-1
      settings: Save2DSignal=2-D array (concatenate along first dimension)
  To Workspace2 : ToWorkspace  VariableName=theta_hat  SampleTime=-1
      settings: Save2DSignal=2-D array (concatenate along first dimension)
  To Workspace3 : ToWorkspace  VariableName=psi_hat  SampleTime=-1
      settings: Save2DSignal=2-D array (concatenate along first dimension)
  To Workspace7 : ToWorkspace  VariableName=phi_true  SampleTime=-1
      settings: Save2DSignal=2-D array (concatenate along first dimension)
  To Workspace8 : ToWorkspace  VariableName=theta_true  SampleTime=-1
      settings: Save2DSignal=2-D array (concatenate along first dimension)
  To Workspace9 : ToWorkspace  VariableName=psi_true  SampleTime=-1
      settings: Save2DSignal=2-D array (concatenate along first dimension)
  phi_true : Outport
  phi_hat : Outport  Port=2
  theta_true : Outport  Port=3
  theta_hat : Outport  Port=4
  psi_true : Outport  Port=5
  psi_hat : Outport  Port=6
  wires:
  A_true/1 -> Radians to Degrees3/1
  Radians to Degrees3/1 -> Demux6/1
  Demux6/1 -> To Workspace7/1, phi_true/1  "phi_mes"
  Demux6/3 -> To Workspace9/1, psi_true/1  "psi_mes"
  Demux6/2 -> To Workspace8/1, theta_true/1  "theta_mes"
  Radians to Degrees1/1 -> Demux1/1
  xhat/1 -> Radians to Degrees1/1
  Demux1/1 -> To Workspace1/1, phi_hat/1  "phi_hat"
  Demux1/3 -> To Workspace3/1, psi_hat/1  "psi_hat"
  Demux1/2 -> To Workspace2/1, theta_hat/1  "theta_hat"

== system ModelAided_PAHRS/AHRS/AHRS (Euler - KF - Closed Loop)/KF ==
  omega_B : Inport
  x_prop : Inport  Port=2
  y_mes : Inport  Port=3
  Enable : EnablePort
  Kalman : MATLAB Function  TreatAsAtomicUnit=on
  deltaxhat : Outport
  wires:
  y_mes/1 -> Kalman/3(y_mes)
  x_prop/1 -> Kalman/2(x_prop)
  omega_B/1 -> Kalman/1(omega_B)
  Kalman/1(deltaxhat) -> deltaxhat/1

== system ModelAided_PAHRS/AHRS/AHRS (Euler - KF - Closed Loop)/Measurement ==
  a_B : Inport
  f_B : Inport  Port=2
  psi_mes : Inport  Port=3
  Measurement : MATLAB Function  TreatAsAtomicUnit=on
  Mux : Mux  Inputs=3
  y_mes : Outport
  wires:
  a_B/1 -> Measurement/1(a_B)
  f_B/1 -> Measurement/2(f_B)
  Mux/1 -> y_mes/1  "y_m"
  psi_mes/1 -> Measurement/3("psi_mes ")
  Measurement/3(psi_mes) -> Mux/3
  Measurement/2(theta_mes) -> Mux/2
  Measurement/1(phi_mes) -> Mux/1

== system ModelAided_PAHRS/AHRS/AHRS (Euler - KF - Closed Loop)/Propagation ==
  omega_B : Inport
  xhat : Inport  Port=2
  Propagation : MATLAB Function  TreatAsAtomicUnit=on
  Unit Delay : UnitDelay  InitialCondition=[0;0;0]  SampleTime=-1  HasFrameUpgradeWarning=on
  x_prop : Outport
  wires:
  xhat/1 -> Unit Delay/1
  Unit Delay/1 -> Propagation/2(Ahat)
  omega_B/1 -> Propagation/1(omega_B)
  Propagation/1(A_prop) -> x_prop/1

== system ModelAided_PAHRS/AHRS/Dynamic Model/Controller ==
  h : Inport
  phi : Inport  Port=2
  theta : Inport  Port=3
  psi : Inport  Port=4
  Clock : Clock
  MATLAB Function : MATLAB Function  TreatAsAtomicUnit=on
  h Controller : Subsystem
  hd : Constant  Value=10  SampleTime=-1
  phi Controller : Subsystem
  psi Controller : Subsystem
  theta Controller : Subsystem
  u1 : Outport
  u2 : Outport  Port=2
  u3 : Outport  Port=3
  u4 : Outport  Port=4
  wires:
  MATLAB Function/3(psid) -> psi Controller/2(psid)
  hd/1 -> h Controller/4(hd)
  psi/1 -> psi Controller/1(psi)  "psi"
  theta Controller/1(u3) -> u3/1
  h/1 -> h Controller/1(h)
  Clock/1 -> MATLAB Function/1(t)
  MATLAB Function/2(thetad) -> theta Controller/2(thetad)
  theta/1 -> h Controller/3(theta), theta Controller/1(theta)  "theta"
  phi Controller/1(u2) -> u2/1
  h Controller/1(u1) -> u1/1
  psi Controller/1(u4) -> u4/1
  phi/1 -> h Controller/2(phi), phi Controller/1(phi)  "phi"
  MATLAB Function/1(phid) -> phi Controller/2(phid)

== system ModelAided_PAHRS/Gravity/Dynamic Model/Controller ==
  h : Inport
  phi : Inport  Port=2
  theta : Inport  Port=3
  psi : Inport  Port=4
  Clock : Clock
  MATLAB Function : MATLAB Function  TreatAsAtomicUnit=on
  h Controller : Subsystem
  hd : Constant  Value=10  SampleTime=-1
  phi Controller : Subsystem
  psi Controller : Subsystem
  theta Controller : Subsystem
  u1 : Outport
  u2 : Outport  Port=2
  u3 : Outport  Port=3
  u4 : Outport  Port=4
  wires:
  MATLAB Function/3(psid) -> psi Controller/2(psid)
  hd/1 -> h Controller/4(hd)
  psi/1 -> psi Controller/1(psi)  "psi"
  theta Controller/1(u3) -> u3/1
  h/1 -> h Controller/1(h)
  Clock/1 -> MATLAB Function/1(t)
  MATLAB Function/2(thetad) -> theta Controller/2(thetad)
  theta/1 -> h Controller/3(theta), theta Controller/1(theta)  "theta"
  phi Controller/1(u2) -> u2/1
  h Controller/1(u1) -> u1/1
  psi Controller/1(u4) -> u4/1
  phi/1 -> h Controller/2(phi), phi Controller/1(phi)  "phi"
  MATLAB Function/1(phid) -> phi Controller/2(phid)

== system ModelAided_PAHRS/Gravity/PAHRS (Euler - KF - Closed Loop)/KF1 ==
  omega_B : Inport
  x_prop : Inport  Port=2
  y_mes1 : Inport  Port=3
  Enable : EnablePort
  Kalman : MATLAB Function  TreatAsAtomicUnit=on
  deltaxhat1 : Outport
  wires:
  y_mes1/1 -> Kalman/3(y_mes)
  x_prop/1 -> Kalman/2(x_prop)
  omega_B/1 -> Kalman/1(omega_B)
  Kalman/1(deltaxhat) -> deltaxhat1/1

== system ModelAided_PAHRS/Gravity/PAHRS (Euler - KF - Closed Loop)/KF2 ==
  omega_B : Inport
  x_prop : Inport  Port=2
  y_mes2 : Inport  Port=3
  Enable : EnablePort
  Kalman : MATLAB Function  TreatAsAtomicUnit=on
  deltaxhat2 : Outport
  wires:
  Kalman/1(deltaxhat) -> deltaxhat2/1
  omega_B/1 -> Kalman/1(omega_B)
  x_prop/1 -> Kalman/2(x_prop)
  y_mes2/1 -> Kalman/3(y_mes)

== system ModelAided_PAHRS/Gravity/PAHRS (Euler - KF - Closed Loop)/Measurement ==
  a_B : Inport
  f_B : Inport  Port=2
  psi_mes1 : Inport  Port=3
  psi_mes2 : Inport  Port=4
  xhat : Inport  Port=5
  Measurement : MATLAB Function  TreatAsAtomicUnit=on
  Mux : Mux  Inputs=2
  Unit Delay : UnitDelay  InitialCondition=[0;0;0]  SampleTime=-1  HasFrameUpgradeWarning=on
  psi_mes : MATLAB Function  TreatAsAtomicUnit=on
  y_mes1 : Outport
  y_mes2 : Outport  Port=2
  wires:
  Measurement/1(phi_mes) -> Mux/1
  Measurement/2(theta_mes) -> Mux/2
  Mux/1 -> y_mes1/1  "y_m"
  f_B/1 -> Measurement/2(f_B)
  a_B/1 -> Measurement/1(a_B)
  xhat/1 -> Unit Delay/1
  Unit Delay/1 -> psi_mes/3(xhat)
  psi_mes2/1 -> psi_mes/2(psi_mes2)
  psi_mes1/1 -> psi_mes/1(psi_mes1)
  psi_mes/1(y_mes2) -> y_mes2/1

== system ModelAided_PAHRS/Gravity/PAHRS (Euler - KF - Closed Loop)/Propagation ==
  omega_B : Inport
  xhat : Inport  Port=2
  Propagation : MATLAB Function  TreatAsAtomicUnit=on
  Unit Delay : UnitDelay  InitialCondition=[0;0;0]  SampleTime=-1  HasFrameUpgradeWarning=on
  x_prop : Outport
  wires:
  Propagation/1(A_prop) -> x_prop/1
  xhat/1 -> Unit Delay/1
  Unit Delay/1 -> Propagation/2(Ahat)
  omega_B/1 -> Propagation/1(omega_B)

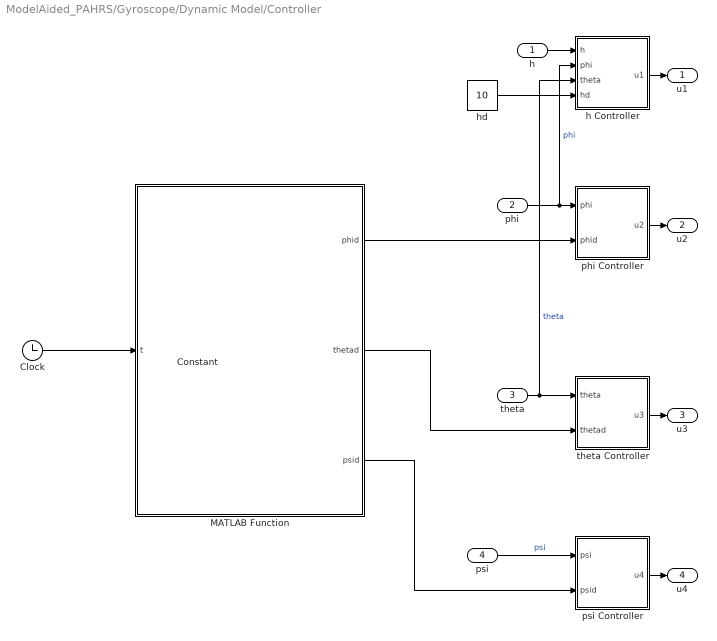
== system ModelAided_PAHRS/Gyroscope/Dynamic Model/Controller ==
  h : Inport
  phi : Inport  Port=2
  theta : Inport  Port=3
  psi : Inport  Port=4
  Clock : Clock
  Constant : Constant
  MATLAB Function : MATLAB Function  TreatAsAtomicUnit=on
  h Controller : Subsystem
  hd : Constant  Value=10  SampleTime=-1
  phi Controller : Subsystem
  psi Controller : Subsystem
  theta Controller : Subsystem
  u1 : Outport
  u2 : Outport  Port=2
  u3 : Outport  Port=3
  u4 : Outport  Port=4
  wires:
  MATLAB Function/3(psid) -> psi Controller/2(psid)
  hd/1 -> h Controller/4(hd)
  psi/1 -> psi Controller/1(psi)  "psi"
  theta Controller/1(u3) -> u3/1
  h/1 -> h Controller/1(h)
  Clock/1 -> MATLAB Function/1(t)
  MATLAB Function/2(thetad) -> theta Controller/2(thetad)
  theta/1 -> h Controller/3(theta), theta Controller/1(theta)  "theta"
  phi Controller/1(u2) -> u2/1
  h Controller/1(u1) -> u1/1
  psi Controller/1(u4) -> u4/1
  phi/1 -> h Controller/2(phi), phi Controller/1(phi)  "phi"
  MATLAB Function/1(phid) -> phi Controller/2(phid)

== system ModelAided_PAHRS/PAHRS/Dynamic Model/Controller ==
  h : Inport
  phi : Inport  Port=2
  theta : Inport  Port=3
  psi : Inport  Port=4
  Clock : Clock
  MATLAB Function : MATLAB Function  TreatAsAtomicUnit=on
  h Controller : Subsystem
  hd : Constant  Value=10  SampleTime=-1
  phi Controller : Subsystem
  psi Controller : Subsystem
  theta Controller : Subsystem
  u1 : Outport
  u2 : Outport  Port=2
  u3 : Outport  Port=3
  u4 : Outport  Port=4
  wires:
  MATLAB Function/3(psid) -> psi Controller/2(psid)
  hd/1 -> h Controller/4(hd)
  psi/1 -> psi Controller/1(psi)  "psi"
  theta Controller/1(u3) -> u3/1
  h/1 -> h Controller/1(h)
  Clock/1 -> MATLAB Function/1(t)
  MATLAB Function/2(thetad) -> theta Controller/2(thetad)
  theta/1 -> h Controller/3(theta), theta Controller/1(theta)  "theta"
  phi Controller/1(u2) -> u2/1
  h Controller/1(u1) -> u1/1
  psi Controller/1(u4) -> u4/1
  phi/1 -> h Controller/2(phi), phi Controller/1(phi)  "phi"
  MATLAB Function/1(phid) -> phi Controller/2(phid)

== system ModelAided_PAHRS/PAHRS/PAHRS (Euler - KF - Closed Loop)/KF1 ==
  omega_B : Inport
  x_prop : Inport  Port=2
  y_mes1 : Inport  Port=3
  Enable : EnablePort
  Kalman : MATLAB Function  TreatAsAtomicUnit=on
  deltaxhat1 : Outport
  wires:
  Kalman/1(deltaxhat) -> deltaxhat1/1
  omega_B/1 -> Kalman/1(omega_B)
  x_prop/1 -> Kalman/2(x_prop)
  y_mes1/1 -> Kalman/3(y_mes)

== system ModelAided_PAHRS/PAHRS/PAHRS (Euler - KF - Closed Loop)/KF2 ==
  omega_B : Inport
  x_prop : Inport  Port=2
  y_mes2 : Inport  Port=3
  Enable : EnablePort
  Kalman : MATLAB Function  TreatAsAtomicUnit=on
  deltaxhat2 : Outport
  wires:
  y_mes2/1 -> Kalman/3(y_mes)
  x_prop/1 -> Kalman/2(x_prop)
  omega_B/1 -> Kalman/1(omega_B)
  Kalman/1(deltaxhat) -> deltaxhat2/1

== system ModelAided_PAHRS/PAHRS/PAHRS (Euler - KF - Closed Loop)/Measurement ==
  a_B : Inport
  f_B : Inport  Port=2
  psi_mes1 : Inport  Port=3
  psi_mes2 : Inport  Port=4
  xhat : Inport  Port=5
  Measurement : MATLAB Function  TreatAsAtomicUnit=on
  Mux : Mux  Inputs=2
  Unit Delay : UnitDelay  InitialCondition=[0;0;0]  SampleTime=-1  HasFrameUpgradeWarning=on
  psi_mes : MATLAB Function  TreatAsAtomicUnit=on
  y_mes1 : Outport
  y_mes2 : Outport  Port=2
  wires:
  Measurement/1(phi_mes) -> Mux/1
  Measurement/2(theta_mes) -> Mux/2
  Mux/1 -> y_mes1/1  "y_m"
  f_B/1 -> Measurement/2(f_B)
  a_B/1 -> Measurement/1(a_B)
  xhat/1 -> Unit Delay/1
  Unit Delay/1 -> psi_mes/3(xhat)
  psi_mes2/1 -> psi_mes/2(psi_mes2)
  psi_mes1/1 -> psi_mes/1(psi_mes1)
  psi_mes/1(y_mes2) -> y_mes2/1

== system ModelAided_PAHRS/PAHRS/PAHRS (Euler - KF - Closed Loop)/Propagation ==
  omega_B : Inport
  xhat : Inport  Port=2
  Propagation : MATLAB Function  TreatAsAtomicUnit=on
  Unit Delay : UnitDelay  InitialCondition=[0;0;0]  SampleTime=-1  HasFrameUpgradeWarning=on
  x_prop : Outport
  wires:
  omega_B/1 -> Propagation/1(omega_B)
  Unit Delay/1 -> Propagation/2(Ahat)
  xhat/1 -> Unit Delay/1
  Propagation/1(A_prop) -> x_prop/1

== system ModelAided_PAHRS/AHRS/Dynamic Model/Controller/h Controller ==
  h : Inport
  phi : Inport  Port=2
  theta : Inport  Port=3
  hd : Inport  Port=4
  Add : Sum
  PID Controller : slpidlib/PID Controller  Controller=PID  Form=Parallel  TimeDomain=Continuous-time  UseExternalTs=off  SampleTime=-1  IntegratorMethod=Forward Euler  FilterMethod=Forward Euler  ControllerParametersSource=internal  P=0.062388232461015  I=0.0029206912699294  UseKiTs=off  D=0.327237449827022  UseExternalDerivativeSource=off  N=5.45397025421619  UseFilter=on  TunerSelectOption=Transfer Function Based (PID Tuner App)  InitialConditionSource=internal  InitialConditionForIntegrator=0  InitialConditionForFilter=0  DifferentiatorICPrevScaledInput=0  ExternalReset=none  TrackingMode=off  Kt=1  LimitOutput=off  SatLimitsSource=internal  UpperSaturationLimit=inf  LowerSaturationLimit=-inf  LinearizeAsGain=on  AntiWindupMode=none  Kb=1  LimitIntegrator=off  UpperIntegratorSaturationLimit=inf  LowerIntegratorSaturationLimit=-inf  POutMin=[]  POutMax=[]  IOutMin=[]  IOutMax=[]  DOutMin=[]  DOutMax=[]  NOutMin=[]  NOutMax=[]  SumOutMin=[]  SumOutMax=[]  SaturationOutMin=[]  SaturationOutMax=[]  PParamMin=[]  PParamMax=[]  IParamMin=[]  IParamMax=[]  DParamMin=[]  DParamMax=[]  NParamMin=[]  NParamMax=[]  KbParamMin=[]  KbParamMax=[]  KtParamMin=[]  KtParamMax=[]  KbOutMin=[]  KbOutMax=[]  KtOutMin=[]  KtOutMax=[]  IntegratorOutMin=[]  IntegratorOutMax=[]  FilterOutMin=[]  FilterOutMax=[]  SumI1OutMin=[]  SumI1OutMax=[]  SumI2OutMin=[]  SumI2OutMax=[]  SumI3OutMin=[]  SumI3OutMax=[]  SumI4OutMin=[]  SumI4OutMax=[]  SumDOutMin=[]  SumDOutMax=[]  DifferentiatorOutMin=[]  DifferentiatorOutMax=[]  FilterDiffOutCoefMin=[]  FilterDiffOutCoefMax=[]  ReciprocalOutMin=[]  ReciprocalOutMax=[]  SumDenOutMin=[]  SumDenOutMax=[]  SumNumOutMin=[]  SumNumOutMax=[]  DivideOutMin=[]  DivideOutMax=[]  UdiffTsProdOutMin=[]  UdiffTsProdOutMax=[]  NTsProdOutMin=[]  NTsProdOutMax=[]  UintegralTsProdOutMin=[]  UintegralTsProdOutMax=[]  UngainTsProdOutMin=[]  UngainTsProdOutMax=[]  ClampingZeroOutDataTypeStr=Inherit: Inherit via back propagation  ClampingZeroOutMin=[]  ClampingZeroOutMax=[]  FilterDenConstantOutDataTypeStr=Inherit: Inherit via back propagation  FilterDenConstantOutMin=[]  FilterDenConstantOutMax=[]  PCopyOutDataTypeStr=Inherit: Inherit via back propagation  PCopyOutMin=[]  PCopyOutMax=[]  NCopyOutDataTypeStr=Inherit: Inherit via back propagation  NCopyOutMin=[]  NCopyOutMax=[]  IntegratorContinuousStateAttributes=''  IntegratorStateMustResolveToSignalObject=off  IntegratorRTWStateStorageClass=Auto  FilterContinuousStateAttributes=''  FilterStateMustResolveToSignalObject=off  FilterRTWStateStorageClass=Auto  ParallelPVariant=InternalParameters  IdealPVariant=Disabled  IVariant=InternalParameters  DVariant=InternalParameters  IntegratorVariant=Continuous  SatVariant=Disabled  AWVariant=Passthrough  PCopyVariant=Disabled  TRVariant=Disabled  FdbkBlocksVariant=Forward  IdealPFdbkVariant=Disabled  SatFdbkVariant=Disabled  DerivativeFilterVariant=ContFilter  NVariant=InternalParameters  NCopyVariant=Disabled  FilterICVariant=InternalICsFilter  IntegratorICVariant=InternalICs  ExternalResetVariant=Disabled  TRSumVariant=Passthrough  SumFdbkVariant=Disabled  SumVariant=Sum_PID  TsampFilterVariant=InternalTs  TsampNgainVariant=Passthrough  TsampIntegralVariant=Disabled_SignalSpec  ExternalSaturationOutDataTypeStr=Inherit: Same as second input  DerivativeSourceVariant=ErrorSignal  PreIntVariant=InternalPreInt
  Sum : Sum  Inputs=|+-
  ustar : MATLAB Function  TreatAsAtomicUnit=on
  u1 : Outport
  wires:
  Sum/1 -> PID Controller/1
  PID Controller/1 -> Add/1  "u1"
  Add/1 -> u1/1
  ustar/1(ustar) -> Add/2
  hd/1 -> Sum/1
  phi/1 -> ustar/1(phi)
  theta/1 -> ustar/2(theta)
  h/1 -> Sum/2

== system ModelAided_PAHRS/AHRS/Dynamic Model/Controller/phi Controller ==
  phi : Inport
  phid : Inport  Port=2
  PID Controller : slpidlib/PID Controller  Controller=PID  Form=Parallel  TimeDomain=Continuous-time  UseExternalTs=off  SampleTime=-1  IntegratorMethod=Forward Euler  FilterMethod=Forward Euler  ControllerParametersSource=internal  P=0.000241576335651922  I=5.32043472864589e-06  UseKiTs=off  D=0.00267047548389725  UseExternalDerivativeSource=off  N=62.8030684622843  UseFilter=on  TunerSelectOption=Transfer Function Based (PID Tuner App)  InitialConditionSource=internal  InitialConditionForIntegrator=0  InitialConditionForFilter=0  DifferentiatorICPrevScaledInput=0  ExternalReset=none  TrackingMode=off  Kt=1  LimitOutput=off  SatLimitsSource=internal  UpperSaturationLimit=inf  LowerSaturationLimit=-inf  LinearizeAsGain=on  AntiWindupMode=none  Kb=1  LimitIntegrator=off  UpperIntegratorSaturationLimit=inf  LowerIntegratorSaturationLimit=-inf  POutMin=[]  POutMax=[]  IOutMin=[]  IOutMax=[]  DOutMin=[]  DOutMax=[]  NOutMin=[]  NOutMax=[]  SumOutMin=[]  SumOutMax=[]  SaturationOutMin=[]  SaturationOutMax=[]  PParamMin=[]  PParamMax=[]  IParamMin=[]  IParamMax=[]  DParamMin=[]  DParamMax=[]  NParamMin=[]  NParamMax=[]  KbParamMin=[]  KbParamMax=[]  KtParamMin=[]  KtParamMax=[]  KbOutMin=[]  KbOutMax=[]  KtOutMin=[]  KtOutMax=[]  IntegratorOutMin=[]  IntegratorOutMax=[]  FilterOutMin=[]  FilterOutMax=[]  SumI1OutMin=[]  SumI1OutMax=[]  SumI2OutMin=[]  SumI2OutMax=[]  SumI3OutMin=[]  SumI3OutMax=[]  SumI4OutMin=[]  SumI4OutMax=[]  SumDOutMin=[]  SumDOutMax=[]  DifferentiatorOutMin=[]  DifferentiatorOutMax=[]  FilterDiffOutCoefMin=[]  FilterDiffOutCoefMax=[]  ReciprocalOutMin=[]  ReciprocalOutMax=[]  SumDenOutMin=[]  SumDenOutMax=[]  SumNumOutMin=[]  SumNumOutMax=[]  DivideOutMin=[]  DivideOutMax=[]  UdiffTsProdOutMin=[]  UdiffTsProdOutMax=[]  NTsProdOutMin=[]  NTsProdOutMax=[]  UintegralTsProdOutMin=[]  UintegralTsProdOutMax=[]  UngainTsProdOutMin=[]  UngainTsProdOutMax=[]  ClampingZeroOutDataTypeStr=Inherit: Inherit via back propagation  ClampingZeroOutMin=[]  ClampingZeroOutMax=[]  FilterDenConstantOutDataTypeStr=Inherit: Inherit via back propagation  FilterDenConstantOutMin=[]  FilterDenConstantOutMax=[]  PCopyOutDataTypeStr=Inherit: Inherit via back propagation  PCopyOutMin=[]  PCopyOutMax=[]  NCopyOutDataTypeStr=Inherit: Inherit via back propagation  NCopyOutMin=[]  NCopyOutMax=[]  IntegratorContinuousStateAttributes=''  IntegratorStateMustResolveToSignalObject=off  IntegratorRTWStateStorageClass=Auto  FilterContinuousStateAttributes=''  FilterStateMustResolveToSignalObject=off  FilterRTWStateStorageClass=Auto  ParallelPVariant=InternalParameters  IdealPVariant=Disabled  IVariant=InternalParameters  DVariant=InternalParameters  IntegratorVariant=Continuous  SatVariant=Disabled  AWVariant=Passthrough  PCopyVariant=Disabled  TRVariant=Disabled  FdbkBlocksVariant=Forward  IdealPFdbkVariant=Disabled  SatFdbkVariant=Disabled  DerivativeFilterVariant=ContFilter  NVariant=InternalParameters  NCopyVariant=Disabled  FilterICVariant=InternalICsFilter  IntegratorICVariant=InternalICs  ExternalResetVariant=Disabled  TRSumVariant=Passthrough  SumFdbkVariant=Disabled  SumVariant=Sum_PID  TsampFilterVariant=InternalTs  TsampNgainVariant=Passthrough  TsampIntegralVariant=Disabled_SignalSpec  ExternalSaturationOutDataTypeStr=Inherit: Same as second input  DerivativeSourceVariant=ErrorSignal  PreIntVariant=InternalPreInt
  Sum : Sum  Inputs=|+-
  u2 : Outport
  wires:
  PID Controller/1 -> u2/1  "u2"
  Sum/1 -> PID Controller/1
  phi/1 -> Sum/2
  phid/1 -> Sum/1
